simulink model "Circuito_trifasico_totalmente_controlado"  (R2024a)
settings: Solver=VariableStepAuto  StartTime=0.0  StopTime=10.0  RelTol=1e-3
libraries: spsVoltageMeasurementLib x7, spsThyristorLib x6, spsACVoltageSourceLib x3, spsCurrentMeasurementLib x1, spsSeriesRLCBranchLib x1, spsMultimeterLib x1, spspowerguiLib x1
settings Model: VariantFading=off  Creator=abel  LastModifiedBy=abel

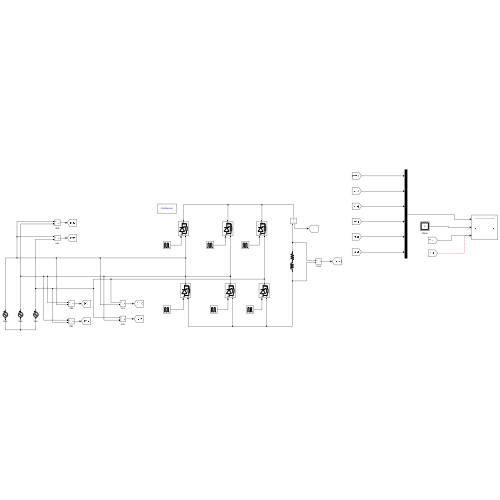
[thumbnail: Simulink's stored preview of the top-level diagram]
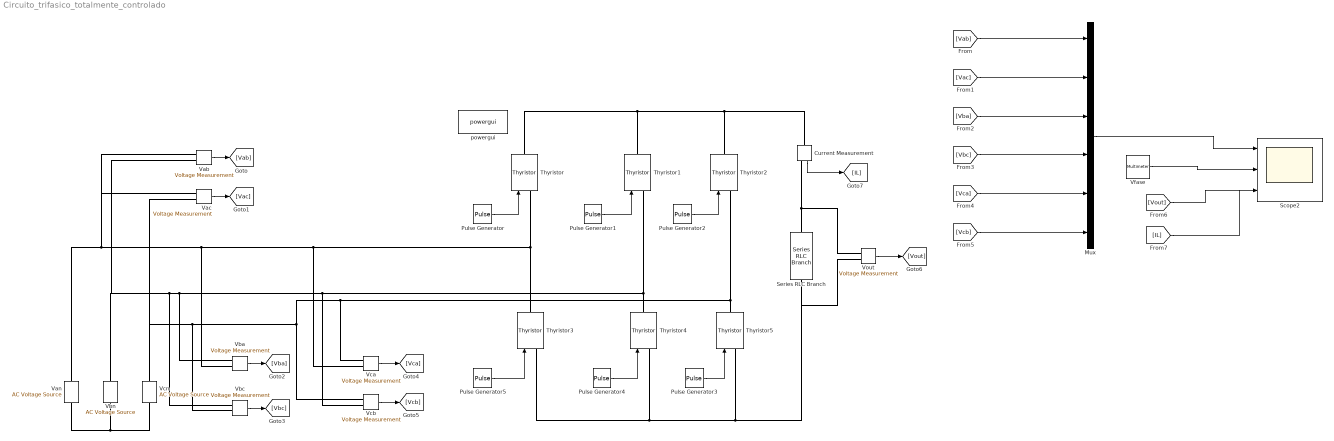
== system Circuito_trifasico_totalmente_controlado ==
  Current Measurement : spsCurrentMeasurementLib/Current Measurement  PhasorSimulation=off  OutputType=Complex  PSBequivalent=0
  Mux : Mux  Inputs=6
  Pulse Generator : DiscretePulseGenerator  PulseType=Time based  Period=0.02  PulseWidth=33.33  PhaseDelay=30*(0.02/360)
  Pulse Generator1 : DiscretePulseGenerator  PulseType=Time based  Period=0.02  PulseWidth=33.3333  PhaseDelay=150*(0.02/360)
  Pulse Generator2 : DiscretePulseGenerator  PulseType=Time based  Period=0.02  PulseWidth=33.3333  PhaseDelay=270*(0.02/360)
  Pulse Generator3 : DiscretePulseGenerator  PulseType=Time based  Period=0.02  PulseWidth=33.3333  PhaseDelay=90*(0.02/360)
  Pulse Generator4 : DiscretePulseGenerator  PulseType=Time based  Period=0.02  PulseWidth=33.3333  PhaseDelay=330*(0.02/360)
  Pulse Generator5 : DiscretePulseGenerator  PulseType=Time based  Period=0.02  PulseWidth=33.3333  PhaseDelay=210*(0.02/360)
  Scope2 : Scope  NumInputPorts=3
  Series RLC Branch : spsSeriesRLCBranchLib/Series RLC Branch  LConnTagsString=__new0  RConnTagsString=__new0  BranchType=RL  Resistance=2.5  Inductance=17.5e-3  SetiL0=off  InitialCurrent=0  Capacitance=1e-6  Setx0=off  InitialVoltage=0  Measurements=Branch voltage and current
  Thyristor{,1..5} (6 alike) : spsThyristorLib/Thyristor  Ron=0.001  Lon=0  Vf=0.8  IC=0  Rs=500  Cs=250e-9  Measurements=off
  Vab : spsVoltageMeasurementLib/Voltage Measurement  PhasorSimulation=off  OutputType=Complex  PSBequivalent=0
  Vac : spsVoltageMeasurementLib/Voltage Measurement  PhasorSimulation=off  OutputType=Complex  PSBequivalent=0
  Van : spsACVoltageSourceLib/AC Voltage Source  Amplitude=118  Phase=0  Frequency=50  SampleTime=0  Measurements=Voltage  BusType=swing  Pref=10e3  Qref=0  Qmin=-inf  Qmax=+inf
  Vba : spsVoltageMeasurementLib/Voltage Measurement  PhasorSimulation=off  OutputType=Complex  PSBequivalent=0
  Vbc : spsVoltageMeasurementLib/Voltage Measurement  PhasorSimulation=off  OutputType=Complex  PSBequivalent=0
  Vbn : spsACVoltageSourceLib/AC Voltage Source  Amplitude=118  Phase=-120  Frequency=50  SampleTime=0  Measurements=Voltage  BusType=swing  Pref=10e3  Qref=0  Qmin=-inf  Qmax=+inf
  Vca : spsVoltageMeasurementLib/Voltage Measurement  PhasorSimulation=off  OutputType=Complex  PSBequivalent=0
  Vcb : spsVoltageMeasurementLib/Voltage Measurement  PhasorSimulation=off  OutputType=Complex  PSBequivalent=0
  Vcn : spsACVoltageSourceLib/AC Voltage Source  Amplitude=118  Phase=-240  Frequency=50  SampleTime=0  Measurements=Voltage  BusType=swing  Pref=10e3  Qref=0  Qmin=-inf  Qmax=+inf
  Vfase : spsMultimeterLib/Multimeter  L=5  sel=[2 3 4]  yselected={}  Gain=[1 1 1]  OutputType=Complex  PlotAtSimulationStop=off  PhasorSimulation=off
  Vout : spsVoltageMeasurementLib/Voltage Measurement  PhasorSimulation=off  OutputType=Complex  PSBequivalent=0
  powergui : spspowerguiLib/powergui  Priority=1  SimulationMode=Continuous  SampleTime=50e-6  frequency=60  Iterations=50  frequencyindice=50  Pbase=100e6  ErrMax=1e-4  UnitsV=kV  UnitsW=MW  buscounter=0  FunctionMessages=off  echomessages=off  EnableUseOfTLC=off  CurrentSourceSwitches=off  DisableSnubberDevices=off  DisableRonSwitches=off  DisableVfSwitches=off  DisplayEquations=off  AutomaticDiscreteSolvers=off  SolverType=Tustin/Backward Euler (TBE)  Interpol=off  ExternalGateDelay=off  methode=off  Ts=100  x0status=blocks  SPID=on  SwTol=0  HookPort=off  NonlinearTolerance=1e-4  nMaxIteration=100  ContinueOnMaxIteration=off  RestoreLinks=warning  ResistiveCurrentMeasurement=off  Frange=[0:2:500]  Ylog=off  Xlog=on  ShowGrid=off  save=off  variable=ZData  structure=0  ZoomFFT=off  StartTime=0.0  cycles=1  DisplayStyle=1  fundamental=60  FreqAxis=off  MaxFrequency=1000  frequencyindicesteady=1  RmsSteady=1  display=off
  wires:
  Pulse Generator/1 -> Thyristor/1
  Pulse Generator5/1 -> Thyristor3/1
  Pulse Generator4/1 -> Thyristor4/1
  Pulse Generator3/1 -> Thyristor5/1
  Pulse Generator1/1 -> Thyristor1/1
  Pulse Generator2/1 -> Thyristor2/1
  Vab/1 -> [Vab]
  Vac/1 -> [Vac]
  Vba/1 -> [Vba]
  Vbc/1 -> [Vbc]
  Vca/1 -> [Vca]
  Vcb/1 -> [Vcb]
  [Vab] -> Mux/1
  [Vac] -> Mux/2
  [Vba] -> Mux/3
  [Vbc] -> Mux/4
  [Vca] -> Mux/5
  [Vcb] -> Mux/6
  Mux/1 -> Scope2/1
  Vout/1 -> [Vout]
  Vfase/1 -> Scope2/2
  [Vout] -> Scope2/3
  Current Measurement/1 -> [IL]
  [IL] -> ?
  connections:
  Thyristor1/LConn1 -- Vcb/LConn2 -- Vbc/LConn1 -- Vbn/RConn1 -- Vab/LConn2 -- Vba/LConn1 -- Thyristor4/RConn1
  Thyristor5/RConn1 -- Vcb/LConn1 -- Vbc/LConn2 -- Vcn/RConn1 -- Vac/LConn2 -- Vca/LConn1 -- Thyristor2/LConn1
  Thyristor3/LConn1 -- Vout/LConn2 -- Series RLC Branch/RConn1 -- Thyristor5/LConn1 -- Thyristor4/LConn1
  Thyristor/RConn1 -- Thyristor1/RConn1 -- Current Measurement/LConn1 -- Thyristor2/RConn1
  Thyristor/LConn1 -- Vca/LConn2 -- Vac/LConn1 -- Vab/LConn1 -- Van/RConn1 -- Vba/LConn2 -- Thyristor3/RConn1
  Vcn/LConn1 -- Van/LConn1 -- Vbn/LConn1
  Series RLC Branch/LConn1 -- Current Measurement/RConn1 -- Vout/LConn1
